simulink model "model"  (R2023b)
settings: Solver=FixedStepAuto  StartTime=0.0  StopTime=50  FixedStep=0.01  RelTol=1e-2  AbsTol=1e-2
undefined symbols (not defined in the file or in its folder): control, dynamique, imu, vent, vr
libraries: dspstat3 x3, simulink x3
settings Model: Creator=pmorin  LastModifiedBy=haoyuan
settings SolverCC: AutoScaleAbsTol=off  AlgebraicLoopSolver=TrustRegion  AutoInsertRateTranBlk=on
settings DataIOCC: LimitDataPoints=on  SaveFormat=Array  SignalLoggingSaveFormat=ModelDataLogs  ReturnWorkspaceOutputs=off
settings OptimizationCC: BooleanDataType=off  ExpressionDepthLimit=2147483647  InitFltsAndDblsToZero=on  LifeSpan=inf
settings DebuggingCC: SaveWithParameterizedLinksMsg=none  UnderspecifiedInitializationDetection=Classic  MergeDetectMultiDrivingBlocksExec=none  SignalResolutionControl=TryResolveAllWithWarning  MultiTaskDSMMsg=warning  MultiTaskCondExecSysMsg=none  FcnCallInpInsideContextMsg=warning  UnconnectedInputMsg=warning  UnconnectedOutputMsg=warning  UnconnectedLineMsg=warning  StateNameClashWarn=warning  SFUnexpectedBacktrackingDiag=warning  SFNoUnconditionalDefaultTransitionDiag=warning  SFExecutionAtInitializationDiag=none  ArithmeticOperatorsInVariantConditions=warning
settings HardwareCC: ProdBitPerPointer=32  ProdBitPerSizeT=32  ProdBitPerPtrDiffT=32  ProdLargestAtomicFloat=None  ProdIntDivRoundTo=Undefined  ProdEndianess=Unspecified  ProdWordSize=32  ProdHWDeviceType=32-bit Generic  TargetUnknown=on
settings ModelReferenceCC: EnableRefExpFcnMdlSchedulingChecks=on  PropagateSignalLabelsOutOfModel=off
settings SFSimCC: SimUseLocalCustomCode=off  CustomCodeUndefinedFunction=UseInterfaceOnly
settings RTWCC: RTWUseLocalCustomCode=off
settings CodeAppCC: StateflowObjectComments=on
settings GRTTargetCC: TargetLangStandard=C89/C90 (ANSI)  ModelReferenceCompliant=off  CompOptLevelCompliant=off  CombineOutputUpdateFcns=off  MatFileLogging=off  GRTInterface=on
settings ConfigComp: CovMetricSettings=dw  CovSaveCumulativeToWorkspaceVar=on  CovSaveSingleToWorkspaceVar=on  CovExternalEMLEnable=off

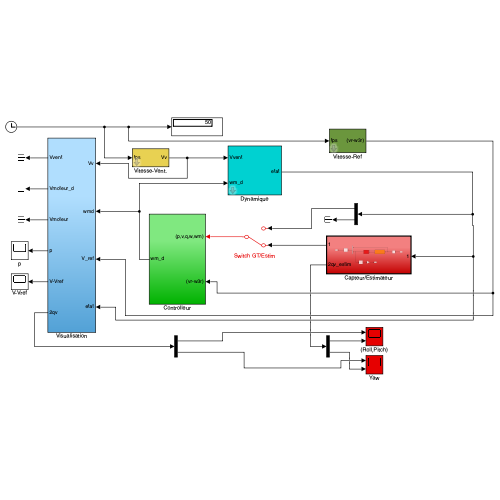
[thumbnail: Simulink's stored preview of the top-level diagram]
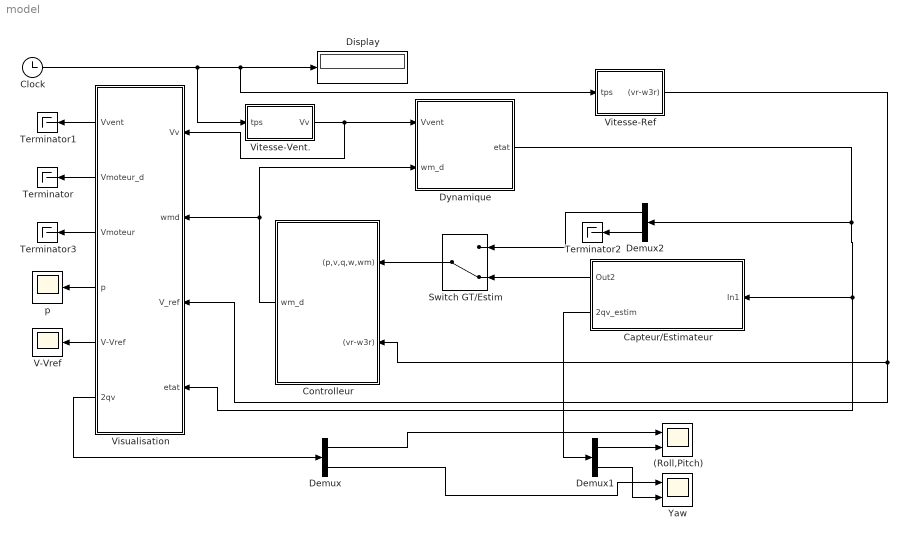
== system model ==
  (Roll,Pitch) : Scope  NumInputPorts=2
  Capteur/Estimateur : Subsystem  TreatAsAtomicUnit=on
  Clock : Clock
  Controlleur : Subsystem
  Demux : Demux  Outputs=[2; 1]
  Demux1 : Demux  Outputs=[2;1]
  Demux2 : Demux  Outputs=[17 3]
  Display : Display
  Dynamique : Subsystem  mask{init=[0.5;0.5;1;0;0;0;sqrt(1-0^2);-0;0;0;0;0;0.3;600;600;600;600]}
      mask prompts: init "Initial values"
  Switch GT/Estim : ManualSwitch  CurrentSetting=0
  Terminator{,1..3} (4 alike) : Terminator
  V-Vref : Scope
  Visualisation : Subsystem
  Vitesse-Ref : Subsystem  mask{choix_traj=Vol non stationnaire}
      mask prompts: choix_traj "trajectoire de reference"
      mask TypeOptions choix_traj: Vol quasi stationnaire | Vol non stationnaire
  Vitesse-Vent. : Subsystem  mask{choix_traj=sans vent}
      mask prompts: choix_traj "trajectoire de reference"
      mask TypeOptions choix_traj: sans vent | vent constant | vent periodique | vent rafale | vent general
  Yaw : Scope  NumInputPorts=2
  p : Scope
  wires:
  Clock/1 -> Vitesse-Vent./1(tps), Vitesse-Ref/1(tps), Display/1
  Vitesse-Vent./1(Vv) -> Visualisation/1(Vv), Dynamique/1(Vvent)
  Controlleur/1(wm_d) -> Dynamique/2(wm_d), Visualisation/2(wmd)
  Visualisation/4(p) -> p/1
  Visualisation/5(V-Vref) -> V-Vref/1
  Visualisation/3("Vmoteur ") -> Terminator3/1
  Vitesse-Ref/1((vr-w3r)) -> Visualisation/3(V_ref), Controlleur/2((vr-w3r))
  Visualisation/2(Vmoteur_d) -> Terminator/1
  Visualisation/1(Vvent) -> Terminator1/1
  Dynamique/1(etat) -> Demux2/1, Visualisation/4(etat), Capteur/Estimateur/1(In1)
  Visualisation/6(2qv) -> Demux/1
  Demux/1 -> (Roll,Pitch)/1
  Demux/2 -> Yaw/1
  Demux1/1 -> (Roll,Pitch)/2
  Demux1/2 -> Yaw/2
  Capteur/Estimateur/2(2qv_estim) -> Demux1/1
  Capteur/Estimateur/1(Out2) -> Switch GT/Estim/2
  Switch GT/Estim/1 -> Controlleur/1((p,v,q,w,wm))
  Demux2/1 -> Switch GT/Estim/1
  Demux2/2 -> Terminator2/1

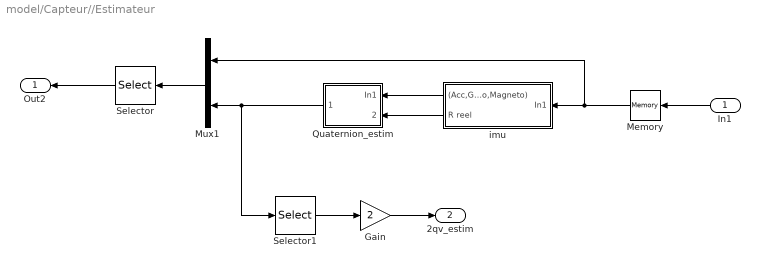
== system model/Capteur//Estimateur ==
  In1 : Inport
  Gain : Gain  Gain=2
  Memory : Memory  InheritSampleTime=on
  Mux1 : Mux  Inputs=2
  Quaternion_estim : Subsystem  TreatAsAtomicUnit=on
  Selector : Selector  InputPortWidth=24  IndexOptions=Index vector (dialog)  Indices=[1 2 3 4 5 6 21 22 23 24 11 12 13 14 15 16 17]  OutputSizes=1
  Selector1 : Selector  InputPortWidth=4  IndexOptions=Index vector (dialog)  Indices=[2 3 4]  OutputSizes=1
  imu : Subsystem  TreatAsAtomicUnit=on
  Out2 : Outport
  2qv_estim : Outport  Port=2
  wires:
  imu/1((Acc,Gyro,Magneto)) -> Quaternion_estim/1(In1)
  Memory/1 -> Mux1/1, imu/1(In1)
  Quaternion_estim/1(q_estim) -> Selector1/1, Mux1/2
  In1/1 -> Memory/1
  Mux1/1 -> Selector/1
  Selector/1 -> Out2/1
  Selector1/1 -> Gain/1
  Gain/1 -> 2qv_estim/1
  imu/2(R reel) -> Quaternion_estim/2(R reel)

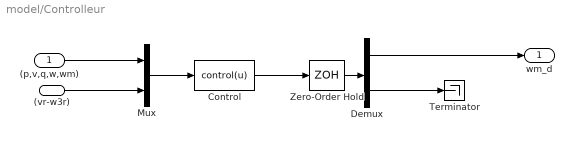
== system model/Controlleur ==
  (p,v,q,w,wm) : Inport
  (vr-w3r) : Inport  Port=2
  Control : MATLABFcn  MATLABFcn=control(u)  OutputDimensions=7
  Demux : Demux  Outputs=2
  Mux : Mux  Inputs=2
  Terminator : Terminator
  Zero-Order Hold : ZeroOrderHold  SampleTime=0.01
  wm_d : Outport  VectorParamsAs1DForOutWhenUnconnected=off
  wires:
  Control/1 -> Zero-Order Hold/1
  Mux/1 -> Control/1
  (p,v,q,w,wm)/1 -> Mux/1
  Zero-Order Hold/1 -> Demux/1
  Demux/1 -> wm_d/1
  Demux/2 -> Terminator/1
  (vr-w3r)/1 -> Mux/2

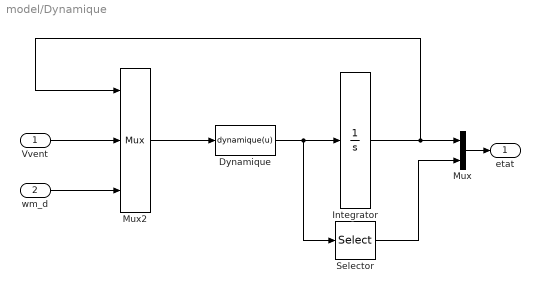
== system model/Dynamique ==
  Vvent : Inport
  wm_d : Inport  Port=2
  Dynamique : MATLABFcn  MATLABFcn=dynamique(u)  OutputDimensions=17
  Integrator : Integrator  InitialCondition=init
  Mux : Mux  Inputs=2
  Mux2 : Mux  Inputs=[17 3 4]
  Selector : Selector  InputPortWidth=17  IndexOptions=Index vector (dialog)  Indices=[4 5 6]  OutputSizes=1
  etat : Outport  VectorParamsAs1DForOutWhenUnconnected=off
  wires:
  Vvent/1 -> Mux2/2
  wm_d/1 -> Mux2/3
  Mux2/1 -> Dynamique/1
  Dynamique/1 -> Selector/1, Integrator/1
  Mux/1 -> etat/1
  Selector/1 -> Mux/2
  Integrator/1 -> Mux2/1, Mux/1

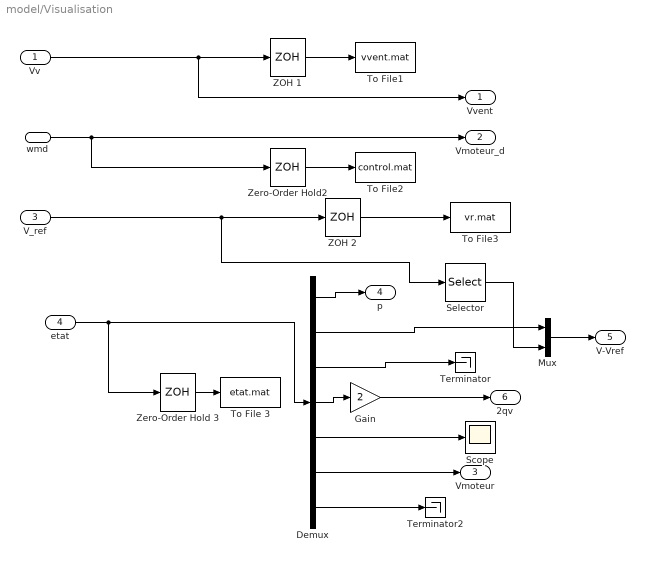
== system model/Visualisation ==
  Vv : Inport
  wmd : Inport  Port=2
  V_ref : Inport  Port=3
  etat : Inport  Port=4
  Demux : Demux  Outputs=[3 3 1 3 3 4 3]
  Gain : Gain  Gain=2
  Mux : Mux  Inputs=2
  Scope : Scope
  Selector : Selector  InputPortWidth=4  IndexOptions=Index vector (dialog)  Indices=[1 2 3]  OutputSizes=1
  Terminator : Terminator
  Terminator2 : Terminator
  To File 3 : ToFile  Filename=etat.mat
  To File1 : ToFile  Filename=vvent.mat
  To File2 : ToFile  Filename=control.mat
  To File3 : ToFile  Filename=vr.mat
  ZOH 1 : ZeroOrderHold  SampleTime=0.02
  "ZOH 2 " : ZeroOrderHold  SampleTime=0.4
  Zero-Order Hold 3 : ZeroOrderHold  SampleTime=0.02
  Zero-Order Hold2 : ZeroOrderHold  SampleTime=0.4
  Vvent : Outport  VectorParamsAs1DForOutWhenUnconnected=off
  Vmoteur_d : Outport  Port=2  VectorParamsAs1DForOutWhenUnconnected=off
  "Vmoteur " : Outport  Port=3  VectorParamsAs1DForOutWhenUnconnected=off
  p : Outport  Port=4  VectorParamsAs1DForOutWhenUnconnected=off
  V-Vref : Outport  Port=5  VectorParamsAs1DForOutWhenUnconnected=off
  2qv : Outport  Port=6  VectorParamsAs1DForOutWhenUnconnected=off
  wires:
  Zero-Order Hold 3/1 -> To File 3/1
  Vv/1 -> Vvent/1, ZOH 1/1
  etat/1 -> Zero-Order Hold 3/1, Demux/1
  Zero-Order Hold2/1 -> To File2/1
  ZOH 1/1 -> To File1/1
  Demux/1 -> p/1
  wmd/1 -> Vmoteur_d/1, Zero-Order Hold2/1
  Gain/1 -> 2qv/1
  Demux/4 -> Gain/1
  Demux/3 -> Terminator/1
  Demux/6 -> "Vmoteur "/1
  V_ref/1 -> Selector/1, "ZOH 2 "/1
  "ZOH 2 "/1 -> To File3/1
  Demux/2 -> Mux/1
  Mux/1 -> V-Vref/1
  Selector/1 -> Mux/2
  Demux/5 -> Scope/1
  Demux/7 -> Terminator2/1

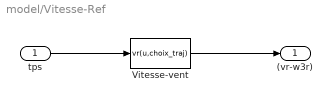
== system model/Vitesse-Ref ==
  tps : Inport
  Vitesse-vent : MATLABFcn  MATLABFcn=vr(u,choix_traj)  OutputDimensions=4
  (vr-w3r) : Outport  VectorParamsAs1DForOutWhenUnconnected=off
  wires:
  Vitesse-vent/1 -> (vr-w3r)/1
  tps/1 -> Vitesse-vent/1

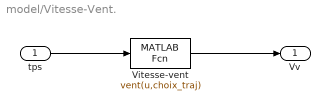
== system model/Vitesse-Vent. ==
  tps : Inport
  Vitesse-vent : MATLABFcn  MATLABFcn=vent(u,choix_traj)  OutputDimensions=3
  Vv : Outport  VectorParamsAs1DForOutWhenUnconnected=off
  wires:
  Vitesse-vent/1 -> Vv/1
  tps/1 -> Vitesse-vent/1

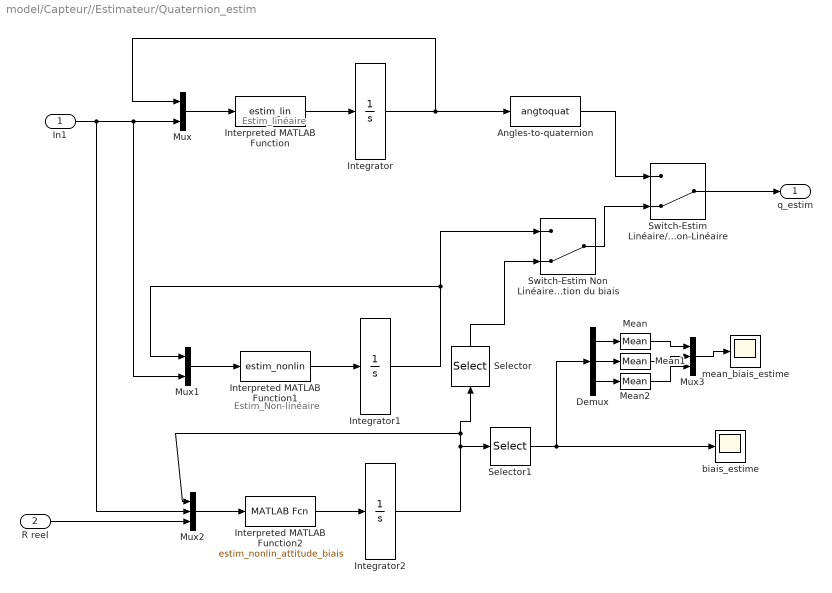
== system model/Capteur//Estimateur/Quaternion_estim ==
  note: Estim_linéaire
  note: Estim_Non-linéaire
  In1 : Inport
  R reel : Inport  Port=2
  Angles-to-quaternion : MATLABFcn  MATLABFcn=angtoquat  OutputDimensions=4
  Demux : Demux  Outputs=3
  Integrator : Integrator  InitialCondition=[0;0;0]
  Integrator1 : Integrator  InitialCondition=[1;0;0;0]
  Integrator2 : Integrator  InitialCondition=[1;0;0;0;0;0;0]
  Interpreted MATLAB Function : MATLABFcn  MATLABFcn=estim_lin  OutputDimensions=3
  Interpreted MATLAB Function1 : MATLABFcn  MATLABFcn=estim_nonlin  OutputDimensions=4
  Interpreted MATLAB Function2 : MATLABFcn  MATLABFcn=estim_nonlin_attitude_biais  OutputDimensions=7
  Mean : dspstat3/Mean  run=on  InputProcessing=Columns as channels (frame based)  reset_popup=None  directionMode=Each column  dimension=1  roiEnable=off  roiType=Rectangles  roiPortion=Entire ROI  roiOutput=Individual statistics for each ROI  roiFlag=off  roundingMode=Floor  overflowMode=off  outputDataTypeStr=Inherit: Same as accumulator  outputMin=[]  outputMax=[]  outputLastDataTypeStr=Inherit: Same as accumulator
  Mean1 : dspstat3/Mean  run=on  InputProcessing=Columns as channels (frame based)  reset_popup=None  directionMode=Each column  dimension=1  roiEnable=off  roiType=Rectangles  roiPortion=Entire ROI  roiOutput=Individual statistics for each ROI  roiFlag=off  roundingMode=Floor  overflowMode=off  outputDataTypeStr=Inherit: Same as accumulator  outputMin=[]  outputMax=[]  outputLastDataTypeStr=Inherit: Same as accumulator
  Mean2 : dspstat3/Mean  run=on  InputProcessing=Columns as channels (frame based)  reset_popup=None  directionMode=Each column  dimension=1  roiEnable=off  roiType=Rectangles  roiPortion=Entire ROI  roiOutput=Individual statistics for each ROI  roiFlag=off  roundingMode=Floor  overflowMode=off  outputDataTypeStr=Inherit: Same as accumulator  outputMin=[]  outputMax=[]  outputLastDataTypeStr=Inherit: Same as accumulator
  Mux : Mux  Inputs=2
  Mux1 : Mux  Inputs=2
  Mux2 : Mux  Inputs=3
  Mux3 : Mux  Inputs=3
  Selector : Selector  InputPortWidth=7  IndexOptions=Index vector (dialog)  Indices=[1 2 3 4]  OutputSizes=1
  Selector1 : Selector  InputPortWidth=7  IndexOptions=Index vector (dialog)  Indices=[5 6 7]  OutputSizes=1
  Switch-Estim Linéaire/Non-Linéaire : ManualSwitch  CurrentSetting=0
  Switch-Estim Non Linéaire normal/Non-Linéaire avec composation du biais : ManualSwitch  CurrentSetting=0
  biais_estime : Scope
  mean_biais_estime : Scope
  q_estim : Outport
  wires:
  In1/1 -> Mux2/2, Mux1/2, Mux/2
  Mux/1 -> Interpreted MATLAB Function/1
  Interpreted MATLAB Function/1 -> Integrator/1
  Integrator/1 -> Angles-to-quaternion/1, Mux/1
  Switch-Estim Linéaire/Non-Linéaire/1 -> q_estim/1
  Interpreted MATLAB Function1/1 -> Integrator1/1
  Mux1/1 -> Interpreted MATLAB Function1/1
  Integrator1/1 -> Mux1/1, Switch-Estim Non Linéaire normal/Non-Linéaire avec composation du biais/1
  Angles-to-quaternion/1 -> Switch-Estim Linéaire/Non-Linéaire/1
  Mux2/1 -> Interpreted MATLAB Function2/1
  Interpreted MATLAB Function2/1 -> Integrator2/1
  Integrator2/1 -> Selector/1, Mux2/1, Selector1/1
  Switch-Estim Non Linéaire normal/Non-Linéaire avec composation du biais/1 -> Switch-Estim Linéaire/Non-Linéaire/2
  R reel/1 -> Mux2/3
  Selector/1 -> Switch-Estim Non Linéaire normal/Non-Linéaire avec composation du biais/2
  Selector1/1 -> biais_estime/1, Demux/1
  Demux/1 -> Mean/1
  Demux/2 -> Mean1/1
  Demux/3 -> Mean2/1
  Mean/1 -> Mux3/1
  Mean1/1 -> Mux3/2
  Mean2/1 -> Mux3/3
  Mux3/1 -> mean_biais_estime/1

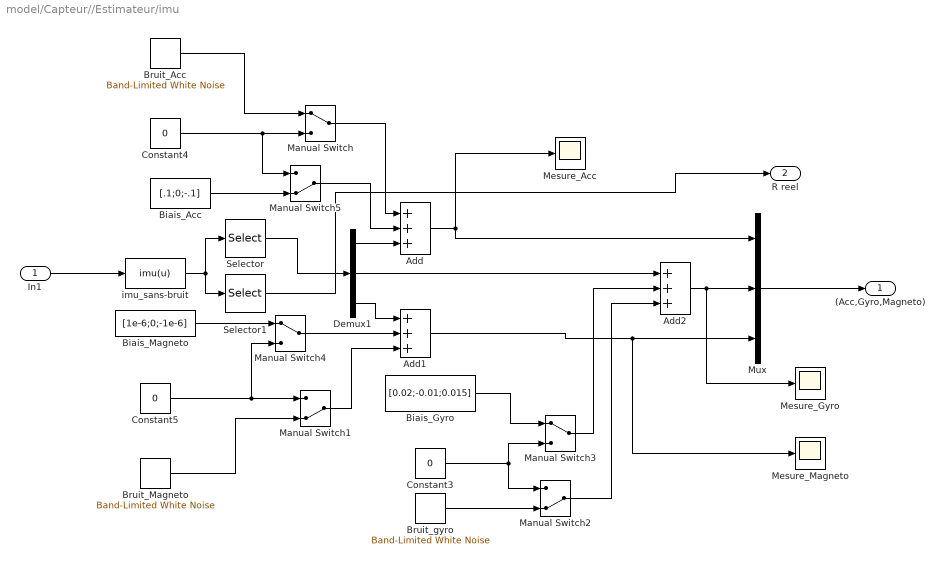
== system model/Capteur//Estimateur/imu ==
  In1 : Inport
  Add : Sum  Inputs=+++
  Add1 : Sum  Inputs=+++
  Add2 : Sum  Inputs=+++
  Biais_Acc : Constant  Value=[.1;0;-.1]
  Biais_Gyro : Constant  Value=[0.02;-0.01;0.015]
  Biais_Magneto : Constant  Value=[1e-6;0;-1e-6]
  Bruit_Acc : simulink/Sources/Band-Limited White Noise  Cov=[0.1]  Ts=0.01  seed=[23341;12025;15426]
  Bruit_Magneto : simulink/Sources/Band-Limited White Noise  Cov=[1e-14]  Ts=0.01  seed=[9821;13120;22478]
  Bruit_gyro : simulink/Sources/Band-Limited White Noise  Cov=[0.001]  Ts=0.01  seed=[21241;15625;17326]
  Constant3 : Constant  Value=0
  Constant4 : Constant  Value=0
  Constant5 : Constant  Value=0
  Demux1 : Demux  Outputs=3
  Manual Switch : ManualSwitch
  Manual Switch1 : ManualSwitch  CurrentSetting=0
  Manual Switch2 : ManualSwitch  CurrentSetting=0
  Manual Switch3 : ManualSwitch
  Manual Switch4 : ManualSwitch
  Manual Switch5 : ManualSwitch  CurrentSetting=0
  Mesure_Acc : Scope
  Mesure_Gyro : Scope
  "Mesure_Magneto " : Scope
  Mux : Mux  Inputs=3
  Selector : Selector  InputPortWidth=18  IndexOptions=Index vector (dialog)  Indices=[1 2 3 4 5 6 7 8 9]  OutputSizes=1
  Selector1 : Selector  InputPortWidth=18  IndexOptions=Index vector (dialog)  Indices=[10 11 12 13 14 15 16 17 18]  OutputSizes=1
  imu_sans-bruit : MATLABFcn  MATLABFcn=imu(u)  OutputDimensions=18
  (Acc,Gyro,Magneto) : Outport  VectorParamsAs1DForOutWhenUnconnected=off
  R reel : Outport  Port=2
  wires:
  In1/1 -> imu_sans-bruit/1
  Add/1 -> Mesure_Acc/1, Mux/1
  Demux1/3 -> Add1/1
  Demux1/2 -> Add2/1
  Add2/1 -> Mesure_Gyro/1, Mux/2
  Add1/1 -> "Mesure_Magneto "/1, Mux/3
  Mux/1 -> (Acc,Gyro,Magneto)/1
  Demux1/1 -> Add/3
  Constant4/1 -> Manual Switch/2, Manual Switch5/1
  Manual Switch/1 -> Add/1
  Manual Switch1/1 -> Add1/3
  Constant5/1 -> Manual Switch4/2, Manual Switch1/1
  Constant3/1 -> Manual Switch2/1, Manual Switch3/2
  Manual Switch2/1 -> Add2/3
  Biais_Gyro/1 -> Manual Switch3/1
  Manual Switch4/1 -> Add1/2
  Biais_Magneto/1 -> Manual Switch4/1
  Manual Switch5/1 -> Add/2
  Biais_Acc/1 -> Manual Switch5/2
  Bruit_Acc/1 -> Manual Switch/1
  Bruit_gyro/1 -> Manual Switch2/2
  Bruit_Magneto/1 -> Manual Switch1/2
  Manual Switch3/1 -> Add2/2
  imu_sans-bruit/1 -> Selector1/1, Selector/1
  Selector/1 -> Demux1/1
  Selector1/1 -> R reel/1
